simulink model "R1_and_P1_Calculation"  (R2024a)
settings: Solver=VariableStepAuto  StartTime=0.0  StopTime=10.0  RelTol=1e-3
settings Model: Creator=ACER  LastModifiedBy=ACER

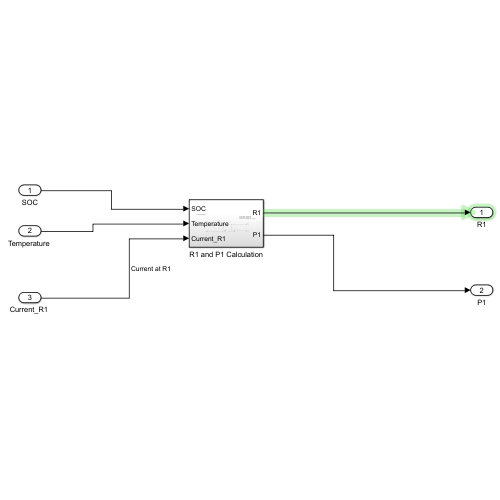
[thumbnail: Simulink's stored preview of the top-level diagram]
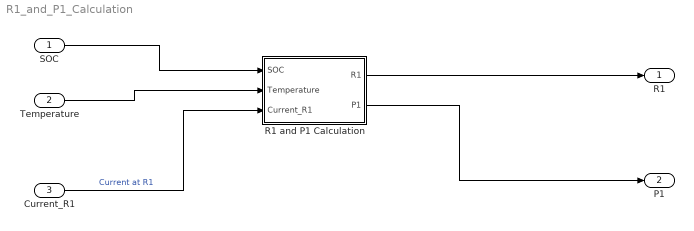
== system R1_and_P1_Calculation ==
  SOC : Inport
  "Temperature " : Inport  Port=2
  "Current_R1 " : Inport  Port=3
  R1 and P1 Calculation : Subsystem
  R1 : Outport
  P1 : Outport  Port=2
  wires:
  SOC/1 -> R1 and P1 Calculation/1(SOC)
  "Temperature "/1 -> R1 and P1 Calculation/2("Temperature ")
  "Current_R1 "/1 -> R1 and P1 Calculation/3("Current_R1 ")  "Current at R1"
  R1 and P1 Calculation/1(R1) -> R1/1
  R1 and P1 Calculation/2(P1) -> P1/1

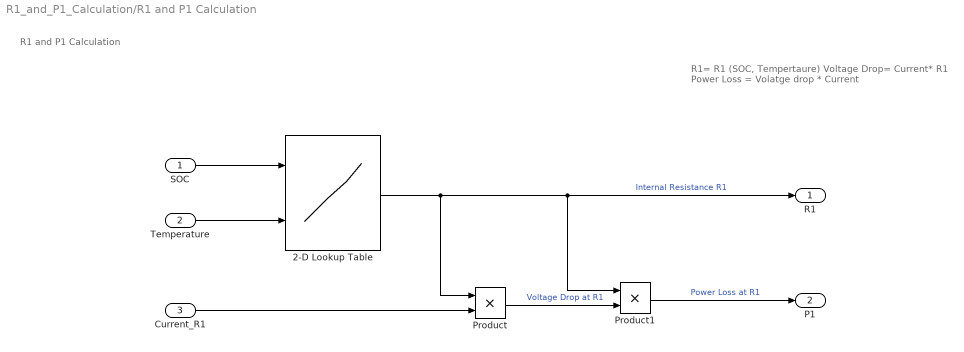
== system R1_and_P1_Calculation/R1 and P1 Calculation ==
  note: R1= R1 (SOC, Tempertaure)
      | Voltage Drop= Current* R1
      | Power Loss = Volatge drop * Current
  note: R1 and P1 Calculation
  SOC : Inport
  "Temperature " : Inport  Port=2
  "Current_R1 " : Inport  Port=3
  2-D Lookup Table : Lookup_n-D  BreakpointsForDimension1=[1:3]  BreakpointsForDimension2=[1:3]  InternalRulePriority=Speed  RndMeth=Simplest
      settings: InputPortMap=u0,u1
  Product : Product
  Product1 : Product
  R1 : Outport
  P1 : Outport  Port=2
  wires:
  SOC/1 -> 2-D Lookup Table/1
  Product1/1 -> P1/1  "Power Loss at R1"
  2-D Lookup Table/1 -> R1/1, Product1/1, Product/1  "Internal Resistance R1"
  Product/1 -> Product1/2  "Voltage Drop at R1"
  "Temperature "/1 -> 2-D Lookup Table/2
  "Current_R1 "/1 -> Product/2
